simulink model "vC_3ph_MR2"  (Simulink 7.9)
settings: Solver=ode14x  StartTime=0.0  StopTime=20/60  FixedStep=Ts1  RelTol=1e-3
PostLoadFcn:
  | , if any(exist('dsrtsu_mdlpostloadfcn', 'file') == [2, 3, 6]), try dsrtsu_mdlpostloadfcn('Execute', bdroot); catch fprintf('Error in PostLoadFcn (dsrtsu_mdlpostloadfcn) for model "%s":\n %s\n', bdroot, lasterr); end, end,
InitFcn:
  | vC_ini
values from neighbouring files (symbols this model uses):
  C = Cideal+deltaC    (= 4e-05)    [IMC_calculo_limites_thetas.m]    (also in IMC_ini.m; JORGE_controlador_LCL_malha_interna.m; LCL_PAPM.m; R_in_LCL.m)
  excitacao_persistente = 0    [iC_ini.m]    (also in vC_ini.m)
  flag_time = 60/60    (= 1)    [iC_ini.m]    (also in vC_ini.m = 0)
  init_time = 60/60    (= 1)    [iC_ini.m]    (also in vC_ini.m)
  L1 = L1ideal+deltaL1    (= 0.002)    [IMC_calculo_limites_thetas.m]    (also in IMC_ini.m; LCL_PAPM.m; R_in_LCL.m; calculo_FTs.m)
  L2 = L2ideal+deltaL2+Lgideal+deltaLg    (= 0.002)    [IMC_calculo_limites_thetas.m]    (also in IMC_ini.m; LCL_PAPM.m; R_in_LCL.m; calculo_FTs.m)
  param_change_time = 60/60    (= 1)    [iC_ini.m]    (also in vC_ini.m)
  R1 = R1ideal+deltaR1    (= 1)    [IMC_calculo_limites_thetas.m]    (also in IMC_ini.m; R_in_LCL.m = 0; gera_resultados.m = 0; iC_ini.m = 0)
  R2 = R2ideal+deltaR2+Rgideal+deltaRg    (= 1)    [IMC_calculo_limites_thetas.m]    (also in IMC_ini.m; R_in_LCL.m = 0; gera_resultados.m = 0; iC_ini.m = 0)
  R_init = 10    [iC_ini.m]    (also in vC_ini.m)
  ref_phaseInv_time = 60/60    (= 1)    [iC_ini.m]    (also in vC_ini.m)
  ref_step_time = 60/60    (= 1)    [iC_ini.m]    (also in vC_ini.m)
  short_OFF_time = 61/60    (= 1.01666666667)    [vC_ini.m]
  short_ON_time = 60/60    (= 1)    [vC_ini.m]
  Ts = 0.5    [IMC_calculo_limites_thetas.m]    (also in IMC_datta_ini.m; IMC_ini.m = 8.33333333333e-05; JORGE_controlador_LCL_malha_interna.m = 8.33333333333e-05; LCL_PAPM.m = 8.33333333333e-05)
  Ts1 = Ts/10    (= 8.33333333333e-06)    [iC_ini.m]    (also in vC_ini.m)
  VCC = 1700    [iC_ini.m]    (also in vC_ini.m = 1200)
undefined symbols (not defined in the file or in its folder): D1, Delta
libraries: powerlib x38, powerlib_extras x1
(part 3 of 3)

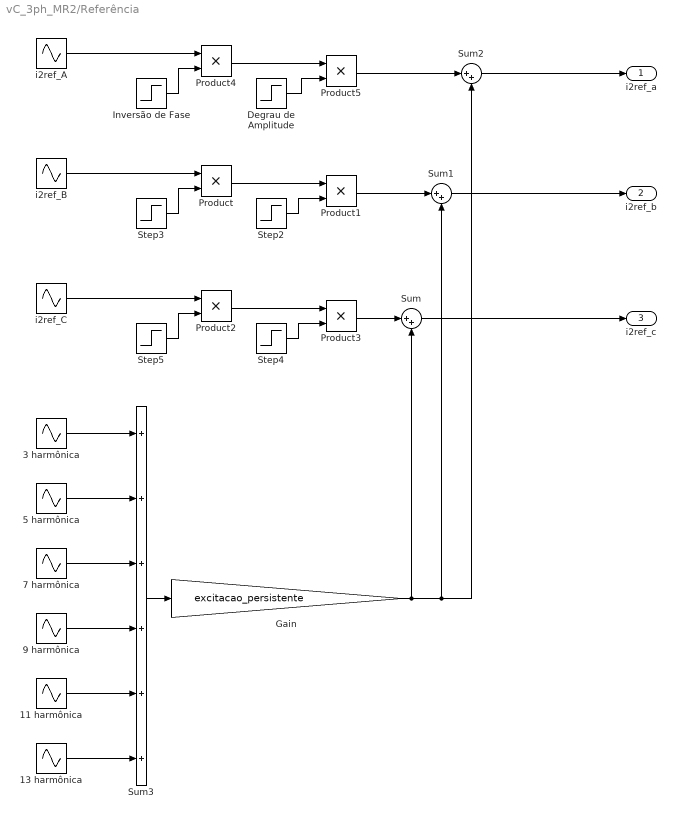
== system vC_3ph_MR2/Referência ==
  11 harmônica : Sin  Amplitude=1.2  Frequency=2*pi*60*11  SampleTime=Ts
  13 harmônica : Sin  Amplitude=1.2  Frequency=2*pi*60*13  SampleTime=Ts
  3 harmônica : Sin  Amplitude=1.2  Frequency=2*pi*60*3  SampleTime=Ts
  5 harmônica : Sin  Amplitude=1.2  Frequency=2*pi*60*5  SampleTime=Ts
  7 harmônica : Sin  Amplitude=1.2  Frequency=2*pi*60*7  SampleTime=Ts
  9 harmônica : Sin  Amplitude=1.2  Frequency=2*pi*60*9  SampleTime=Ts
  Degrau de Amplitude : Step  Time=ref_step_time  Before=1  After=2  SampleTime=Ts
  Gain : Gain  Gain=excitacao_persistente  SampleTime=Ts
  Inversão de Fase : Step  Time=ref_phaseInv_time  Before=1  After=-1  SampleTime=Ts
  Product{,1..5} (6 alike) : Product  SampleTime=Ts  RndMeth=Zero
  Step2 : Step  Time=ref_step_time  Before=1  After=2  SampleTime=Ts
  Step3 : Step  Time=ref_phaseInv_time  Before=1  After=-1  SampleTime=Ts
  Step4 : Step  Time=ref_step_time  Before=1  After=2  SampleTime=Ts
  Step5 : Step  Time=ref_phaseInv_time  Before=1  After=-1  SampleTime=Ts
  Sum : Sum  Inputs=|++
  Sum1 : Sum  Inputs=|++
  Sum2 : Sum  Inputs=|++
  Sum3 : Sum  Inputs=++++++
  i2ref_A : Sin  Amplitude=10  Frequency=2*pi*60  SampleTime=Ts
  i2ref_B : Sin  Amplitude=10  Frequency=2*pi*60  Phase=-2*pi/3  SampleTime=Ts
  i2ref_C : Sin  Amplitude=10  Frequency=2*pi*60  Phase=2*pi/3  SampleTime=Ts
  i2ref_a : Outport
  i2ref_b : Outport  Port=2
  i2ref_c : Outport  Port=3
  wires:
  Product/1 -> Product1/1
  Step3/1 -> Product/2
  Step2/1 -> Product1/2
  Product2/1 -> Product3/1
  Step5/1 -> Product2/2
  Step4/1 -> Product3/2
  Product4/1 -> Product5/1
  Inversão de Fase/1 -> Product4/2
  Degrau de Amplitude/1 -> Product5/2
  i2ref_B/1 -> Product/1
  i2ref_C/1 -> Product2/1
  i2ref_A/1 -> Product4/1
  Product5/1 -> Sum2/1
  Product1/1 -> Sum1/1
  Product3/1 -> Sum/1
  Gain/1 -> Sum/2, Sum1/2, Sum2/2
  Sum2/1 -> i2ref_a/1
  Sum1/1 -> i2ref_b/1
  Sum/1 -> i2ref_c/1
  3 harmônica/1 -> Sum3/1
  5 harmônica/1 -> Sum3/2
  7 harmônica/1 -> Sum3/3
  9 harmônica/1 -> Sum3/4
  11 harmônica/1 -> Sum3/5
  13 harmônica/1 -> Sum3/6
  Sum3/1 -> Gain/1

== matlab function Controlador/abc to alpha-beta-zero ==
  data: i2ref_a input double; i2ref_alpha output double; i2ref_b input double; i2ref_c input double; i2ref_beta output double; i2ref_0 output double
function [i2ref_alpha, i2ref_beta, i2ref_0] = abc2ab0(i2ref_a, i2ref_b, i2ref_c)
%#CODEGEN

alpha_beta_zero = [2/3 -1/3 -1/3; 0 1/sqrt(3) -1/sqrt(3); 1/3 1/3 1/3]*[i2ref_a; i2ref_b; i2ref_c];
%alpha_beta_zero = [0.66666666666667 -0.33333333333333 -0.33333333333333; 0 0.57735026918963 -0.57735026918963; 0.47140452079103 0.47140452079103 0.47140452079103]*[i2ref_a; i2ref_b; i2ref_c];

i2ref_alpha = alpha_beta_zero(1);
i2ref_beta = alpha_beta_zero(2);
i2ref_0 = alpha_beta_zero(3);

== matlab function Controlador/Controlador Adaptativo Alpha ==
  data: i2ref_k input double; up_alpha output double; i2_k input double; vc_k input double; flag input double; theta_alpha output double; t input double; m output double
function [up_alpha, theta_alpha, m] = adaptativo( i2ref_k, i2_k, vc_k, flag, t )

%#CODEGEN

%Definição dos valores projetados dos elementos do filtro
L1ideal=2e-3;
L2ideal=2e-3;
Lgideal=0;
Cideal=40e-6;
R1ideal=0;
R2ideal=0;
Rgideal=0;

%Definição de erros percentuais para simular variação paramétrica
errL1=0;
errL2=0;
errLg=0;
errC=0;
errR1=0;
errR2=0;
errRg=0;
deltaL1=errL1*L1ideal;
deltaL2=errL2*L2ideal;
deltaLg=errLg*Lgideal;
deltaC=errC*Cideal;
deltaR1=errR1*R1ideal;
deltaR2=errR2*R2ideal;
deltaRg=errRg*Rgideal;

%Definição do valor real medido, incluindo a variação paramétrica
%percentual
L1=L1ideal+deltaL1;
L2=L2ideal+deltaL2+Lgideal+deltaLg;
C=Cideal+deltaC;
R1=R1ideal+deltaR1;
R2=R2ideal+deltaR2+Rgideal+deltaRg;

%Demais elementos
Ts=1/12000;
w=sqrt((L1+L2)/(L1*L2*C));

%Kp é a multiplicação do ganho do controlador da malha interna(kp), do
%ganho da planta(ki) e do ganho da malha externa(kod)
kp_kd=3;
%Kp=0.156891976007044;
Kp=0.001792815465831;

%polos do modelo de referência:
p1=0.2;
p2=0.2;

km=(1-p1)*(1-p2);

%constantes -> gamaD < (1-gama)*km/kp
%gamaD=0.01;
gamaD=0.0098;
gama=0.99;

%delta0=0.99;
delta0=0.8;

%% Variáveis Persistentes e Inicializações

persistent theta_k;
if isempty(theta_k)
    %COM compensação para vg
    %theta_k=[-0.3106; -0.2728; 0.0368; -0.2369; -0.422; -0.2775; -0.7979; 1.786; -0.0008; 0.0003];
    %theta_k=[-0.3106; -0.2728; 0.0368; -0.2369; -0.422; -0.2775; -0.7979; 1.786; 1; 0];
    %theta_k=[-0.40085038; -0.36853743; -0.064251891; -0.4277604154; -0.61214672; -0.46675405; -0.98929343; 1.76426551; 0.17164080; 0.11598547];
    %theta_k=[0;0;0;0;0;0; -0.98929343; 1.76426551; 0.17164080; 0.11598547];
    %theta_k=[-0.071151848470510; -0.470549298500393; -0.993323557655345; 1.762541193804541; 0.118014567931226; 0.108368323169129];
    %theta_k=[-0.46; -0.58; -1.74; 1.73; 0.2; 0.03];
    theta_k=[1; -3.39; -0.18; 12.72; 1; 0];
end

persistent omega_k;
if isempty(omega_k)
    %COM vg
    omega_k=[0; 0; 0; 0; 0; 0];
end

persistent omega_k_1;
if isempty(omega_k_1)
    %COM vg
    omega_k_1=[0; 0; 0; 0; 0; 0];
end

persistent omega_k_2;
if isempty(omega_k_2)
    %COM vg
    omega_k_2=[0; 0; 0; 0; 0; 0];
end

persistent omega_k_3;
if isempty(omega_k_3)
    %COM vg
    omega_k_3=[0; 0; 0; 0; 0; 0];
end

persistent eta_k_1;
if isempty(eta_k_1)
    %COM vg
    eta_k_1=[0; 0; 0; 0; 0; 0];
end

persistent eta_k_2;
if isempty(eta_k_2)
    %COM vg
    eta_k_2=[0; 0; 0; 0; 0; 0];
end

persistent eta_k_3;
if isempty(eta_k_3)
    %COM vg
    eta_k_3=[0; 0; 0; 0; 0; 0];
end

persistent i2m_k_1;
if isempty(i2m_k_1)
    i2m_k_1=0;
end

persistent i2m_k_2;
if isempty(i2m_k_2)
    i2m_k_2=0;
end

persistent i2m_k_3;
if isempty(i2m_k_3)
    i2m_k_3=0;
end

persistent i2ref_k_1;
if isempty(i2ref_k_1)
    i2ref_k_1=0;
end

persistent i2ref_k_2;
if isempty(i2ref_k_2)
    i2ref_k_2=0;
end

persistent i2ref_k_3;
if isempty(i2ref_k_3)
    i2ref_k_3=0;
end

persistent v_k_1;
if isempty(v_k_1)
    v_k_1=0;
end

persistent v_k_2;
if isempty(v_k_2)
    v_k_2=0;
end

persistent v_k_3;
if isempty(v_k_3)
    v_k_3=0;
end

persistent rho_k;
if isempty(rho_k)
    rho_k=Kp/km;
end

persistent m2;
if isempty(m2)
    m2=1;
end

persistent vc_k_1;
if isempty(vc_k_1)
    vc_k_1=0;
end

persistent u_k_1;
if isempty(u_k_1)
    u_k_1=0;
end

persistent u_k_2;
if isempty(u_k_2)
    u_k_2=0;
end

persistent P;
if isempty(P)
    %P=[0.002225441018075 -0.002258665319558 -1.129332659782590e-004 -0.003793046611769; ...
    %    -0.002258665319558 0.149747822133961 -0.042512608892738 0.002487914954665; ...
    %    -1.129332659782590e-004 -0.042512608892738 0.997874369555398 1.243957477280539e-004; ...
    %    -0.003793046611769 0.002487914954665 1.243957477280538e-004 0.754190018333160];
    %P=[0.009712540165252   -0.000020445335620  -0.000026266935611  -0.000037334327242 -0.001161097577207  -0.000971095497459; ...
    %   -0.000020445335620   0.009977400822109  -0.000022631160072  -0.000009984284241 -0.000310511239892   0.000028021469709; ...
    %   -0.000026266935611  -0.000022631160072   0.009976301443788  -0.000009972563160 -0.000310146714255   0.000019062507239; ...
    %   -0.000037334327242  -0.000009984284241  -0.000009972563160   0.009989966652248 -0.000312037115068   0.000004936266851; ...
    %   -0.001161097577207  -0.000310511239892  -0.000310146714255  -0.000312037115068 0.000295645721395   0.000153517899078; ...
    %   -0.000971095497459   0.000028021469709   0.000019062507239   0.000004936266851 0.000153517899078   0.000171767843043];

    P=gamaD*eye(6);
end

persistent gama2;
if isempty(gama2)
    %gama2=0.997899999973786;
    gama2=gama;
end


%% Cálculos

%Ação de controle
omega_k(3)= i2_k;
omega_k(4)= i2ref_k;

%COM vg
omega_k(5)= 311*sin(2*pi*60*t);
omega_k(6)= 311*cos(2*pi*60*t);
%omega_k(5)= 0;
%omega_k(6)= 0;

u_k= theta_k'*omega_k;

%inserindo o controlador proporcional no bloco do adaptativo
up_alpha= kp_kd*(u_k - vc_k) - kp_kd*(u_k_1 - vc_k_1);

eta_k= (p1+p2)*eta_k_1 - p1*p2*eta_k_2 + (1-p1)*(1-p2)*omega_k_2;

i2m_k= (p1+p2)*i2m_k_1 - p1*p2*i2m_k_2 + (1-p1)*(1-p2)*i2ref_k_2;

e1_k= i2_k - i2m_k;

v_k= (p1+p2)*v_k_1 - p1*p2*v_k_2 + (1-p1)*(1-p2)*u_k_2;

q_k= theta_k'*eta_k;

e2_k= -v_k+q_k;

ea_k= e1_k+rho_k*e2_k;

eta2_k = eta_k;
eta2_k(5) = 0;
eta2_k(6) = 0;

if flag==1
    %m2_k= 0.01*eta_k'*eta_k + e2_k^2 + m2;
    m2_k= 0.1*eta2_k'*eta2_k + e2_k^2 + m2;
else
    %m2_k= eta_k'*eta_k + e2_k^2 + m2;
    m2_k= 0.01*eta2_k'*eta2_k + e2_k^2 + m2;
end
%m2_k= m2 + (1+eta_k'*P*eta_k) + gama2*e2_k^2;
m = m2_k;

P= P - (P*eta_k*eta_k'*P)/m2_k;
gama2= gama2 - (gama2^2*e2_k^2)/(m2_k^2);

%Pout=P;
%gama_out=gama2;

%% Atualização

%calcula theta(k+1)
theta_k = theta_k - (gamaD*ea_k/m2_k)*eta_k;
%theta_k = theta_k - (P*ea_k/m2_k)*eta_k;
theta_alpha = theta_k;

%calcula rho(k+1)
rho_k= rho_k - (gama*ea_k*e2_k)/m2_k;

if flag==1
    %m2 = delta0*(m2 - 1) + abs(u_k) + abs(i2_k) + 1;
    m2 = delta0*(m2 - 1) + abs(u_k) + abs(i2_k) + 1;
else
    %m2 = delta0*(m2 - 1) + abs(u_k)^2 + abs(i2_k)^2 + 1;
    m2 = delta0*(m2 - 1) + abs(u_k) + abs(i2_k) + 1;
end

omega_k_3=omega_k_2;
omega_k_2=omega_k_1;
omega_k_1=omega_k;

omega_k(1)=0*omega_k(1) + 1*u_k;
omega_k(2)=0*omega_k(2) + 1*i2_k;

eta_k_3=eta_k_2;
eta_k_2=eta_k_1;
eta_k_1=eta_k;

i2ref_k_3 = i2ref_k_2;
i2ref_k_2 = i2ref_k_1;
i2ref_k_1 = i2ref_k;

i2m_k_3=i2m_k_2;
i2m_k_2=i2m_k_1;
i2m_k_1=i2m_k;

v_k_3=v_k_2;
v_k_2=v_k_1;
v_k_1=v_k;

u_k_2=u_k_1;
u_k_1=u_k;

vc_k_1=vc_k;

end

== matlab function Controlador/Controlador Adaptativo Beta ==
  data: i2ref_k input double; up_beta output double; i2_k input double; vc_k input double; flag input double; t input double; theta_beta output double; m output double
function [up_beta, theta_beta, m] = adaptativo( i2ref_k, i2_k, vc_k, flag, t )

%#CODEGEN

%Definição dos valores projetados dos elementos do filtro
L1ideal=2e-3;
L2ideal=2e-3;
Lgideal=0;
Cideal=40e-6;
R1ideal=0;
R2ideal=0;
Rgideal=0;

%Definição de erros percentuais para simular variação paramétrica
errL1=0;
errL2=0;
errLg=0;
errC=0;
errR1=0;
errR2=0;
errRg=0;
deltaL1=errL1*L1ideal;
deltaL2=errL2*L2ideal;
deltaLg=errLg*Lgideal;
deltaC=errC*Cideal;
deltaR1=errR1*R1ideal;
deltaR2=errR2*R2ideal;
deltaRg=errRg*Rgideal;

%Definição do valor real medido, incluindo a variação paramétrica
%percentual
L1=L1ideal+deltaL1;
L2=L2ideal+deltaL2+Lgideal+deltaLg;
C=Cideal+deltaC;
R1=R1ideal+deltaR1;
R2=R2ideal+deltaR2+Rgideal+deltaRg;

%Demais elementos
Ts=1/12000;
w=sqrt((L1+L2)/(L1*L2*C));

%Kp é a multiplicação do ganho do controlador da malha interna(kp), do
%ganho da planta(ki) e do ganho da malha externa(kod)
kp_kd=3;
%Kp=0.156891976007044;
Kp=0.001792815465831;

%polos do modelo de referência:
p1=0.2;
p2=0.2;

km=(1-p1)*(1-p2);

%constantes -> gamaD < (1-gama)*km/kp
%gamaD=0.01;
gamaD=0.0098;
gama=0.99;

%delta0=0.99;
delta0=0.8;

%% Variáveis Persistentes e Inicializações

persistent theta_k;
if isempty(theta_k)
    %COM compensação para vg
    %theta_k=[-0.3106; -0.2728; 0.0368; -0.2369; -0.422; -0.2775; -0.7979; 1.786; -0.0008; 0.0003];
    %theta_k=[-0.3106; -0.2728; 0.0368; -0.2369; -0.422; -0.2775; -0.7979; 1.786; 1; 0];
    %theta_k=[-0.40085038; -0.36853743; -0.064251891; -0.4277604154; -0.61214672; -0.46675405; -0.98929343; 1.76426551; 0.17164080; 0.11598547];
    %theta_k=[0;0;0;0;0;0; -0.98929343; 1.76426551; 0.17164080; 0.11598547];
    %theta_k=[-0.071151848470510; -0.470549298500393; -0.993323557655345; 1.762541193804541; 0.118014567931226; 0.108368323169129];
    %theta_k=[-0.46; -0.58; -1.74; 1.73; 0.2; 0.03];
    theta_k=[1; -3.39; -0.18; 12.72; 0; 1];
end

persistent omega_k;
if isempty(omega_k)
    %COM vg
    omega_k=[0; 0; 0; 0; 0; 0];
end

persistent omega_k_1;
if isempty(omega_k_1)
    %COM vg
    omega_k_1=[0; 0; 0; 0; 0; 0];
end

persistent omega_k_2;
if isempty(omega_k_2)
    %COM vg
    omega_k_2=[0; 0; 0; 0; 0; 0];
end

persistent omega_k_3;
if isempty(omega_k_3)
    %COM vg
    omega_k_3=[0; 0; 0; 0; 0; 0];
end

persistent eta_k_1;
if isempty(eta_k_1)
    %COM vg
    eta_k_1=[0; 0; 0; 0; 0; 0];
end

persistent eta_k_2;
if isempty(eta_k_2)
    %COM vg
    eta_k_2=[0; 0; 0; 0; 0; 0];
end

persistent eta_k_3;
if isempty(eta_k_3)
    %COM vg
    eta_k_3=[0; 0; 0; 0; 0; 0];
end

persistent i2m_k_1;
if isempty(i2m_k_1)
    i2m_k_1=0;
end

persistent i2m_k_2;
if isempty(i2m_k_2)
    i2m_k_2=0;
end

persistent i2m_k_3;
if isempty(i2m_k_3)
    i2m_k_3=0;
end

persistent i2ref_k_1;
if isempty(i2ref_k_1)
    i2ref_k_1=0;
end

persistent i2ref_k_2;
if isempty(i2ref_k_2)
    i2ref_k_2=0;
end

persistent i2ref_k_3;
if isempty(i2ref_k_3)
    i2ref_k_3=0;
end

persistent v_k_1;
if isempty(v_k_1)
    v_k_1=0;
end

persistent v_k_2;
if isempty(v_k_2)
    v_k_2=0;
end

persistent v_k_3;
if isempty(v_k_3)
    v_k_3=0;
end

persistent rho_k;
if isempty(rho_k)
    rho_k=Kp/km;
end

persistent m2;
if isempty(m2)
    m2=1;
end

persistent vc_k_1;
if isempty(vc_k_1)
    vc_k_1=0;
end

persistent u_k_1;
if isempty(u_k_1)
    u_k_1=0;
end

persistent u_k_2;
if isempty(u_k_2)
    u_k_2=0;
end

persistent P;
if isempty(P)
    %P=[0.002225441018075 -0.002258665319558 -1.129332659782590e-004 -0.003793046611769; ...
    %    -0.002258665319558 0.149747822133961 -0.042512608892738 0.002487914954665; ...
    %    -1.129332659782590e-004 -0.042512608892738 0.997874369555398 1.243957477280539e-004; ...
    %    -0.003793046611769 0.002487914954665 1.243957477280538e-004 0.754190018333160];
    %P=[0.009712540165252   -0.000020445335620  -0.000026266935611  -0.000037334327242 -0.001161097577207  -0.000971095497459; ...
    %   -0.000020445335620   0.009977400822109  -0.000022631160072  -0.000009984284241 -0.000310511239892   0.000028021469709; ...
    %   -0.000026266935611  -0.000022631160072   0.009976301443788  -0.000009972563160 -0.000310146714255   0.000019062507239; ...
    %   -0.000037334327242  -0.000009984284241  -0.000009972563160   0.009989966652248 -0.000312037115068   0.000004936266851; ...
    %   -0.001161097577207  -0.000310511239892  -0.000310146714255  -0.000312037115068 0.000295645721395   0.000153517899078; ...
    %   -0.000971095497459   0.000028021469709   0.000019062507239   0.000004936266851 0.000153517899078   0.000171767843043];

    P=gamaD*eye(6);
end

persistent gama2;
if isempty(gama2)
    %gama2=0.997899999973786;
    gama2=gama;
end


%% Cálculos

%Ação de controle
omega_k(3)= i2_k;
omega_k(4)= i2ref_k;

%COM vg
omega_k(5)= 311*sin(2*pi*60*t);
omega_k(6)= 311*cos(2*pi*60*t);
%omega_k(5)= 0;
%omega_k(6)= 0;

u_k= theta_k'*omega_k;

%inserindo o controlador proporcional no bloco do adaptativo
up_beta= kp_kd*(u_k - vc_k) - kp_kd*(u_k_1 - vc_k_1);

eta_k= (p1+p2)*eta_k_1 - p1*p2*eta_k_2 + (1-p1)*(1-p2)*omega_k_2;

i2m_k= (p1+p2)*i2m_k_1 - p1*p2*i2m_k_2 + (1-p1)*(1-p2)*i2ref_k_2;

e1_k= i2_k - i2m_k;

v_k= (p1+p2)*v_k_1 - p1*p2*v_k_2 + (1-p1)*(1-p2)*u_k_2;

q_k= theta_k'*eta_k;

e2_k= -v_k+q_k;

ea_k= e1_k+rho_k*e2_k;

eta2_k = eta_k;
eta2_k(5) = 0;
eta2_k(6) = 0;

if flag==1
    %m2_k= 0.01*eta_k'*eta_k + e2_k^2 + m2;
    m2_k= 0.1*eta2_k'*eta2_k + e2_k^2 + m2;
else
    %m2_k= eta_k'*eta_k + e2_k^2 + m2;
    m2_k= 0.01*eta2_k'*eta2_k + e2_k^2 + m2;
end
%m2_k= m2 + (1+eta_k'*P*eta_k) + gama2*e2_k^2;
m = m2_k;

P= P - (P*eta_k*eta_k'*P)/m2_k;
gama2= gama2 - (gama2^2*e2_k^2)/(m2_k^2);

%Pout=P;
%gama_out=gama2;

%% Atualização

%calcula theta(k+1)
theta_k = theta_k - (gamaD*ea_k/m2_k)*eta_k;
%theta_k = theta_k - (P*ea_k/m2_k)*eta_k;
theta_beta = theta_k;

%calcula rho(k+1)
rho_k= rho_k - (gama*ea_k*e2_k)/m2_k;

if flag==1
    %m2 = delta0*(m2 - 1) + abs(u_k) + abs(i2_k) + 1;
    m2 = delta0*(m2 - 1) + abs(u_k) + abs(i2_k) + 1;
else
    %m2 = delta0*(m2 - 1) + abs(u_k)^2 + abs(i2_k)^2 + 1;
    m2 = delta0*(m2 - 1) + abs(u_k) + abs(i2_k) + 1;
end

omega_k_3=omega_k_2;
omega_k_2=omega_k_1;
omega_k_1=omega_k;

omega_k(1)=0*omega_k(1) + 1*u_k;
omega_k(2)=0*omega_k(2) + 1*i2_k;

eta_k_3=eta_k_2;
eta_k_2=eta_k_1;
eta_k_1=eta_k;

i2ref_k_3 = i2ref_k_2;
i2ref_k_2 = i2ref_k_1;
i2ref_k_1 = i2ref_k;

i2m_k_3=i2m_k_2;
i2m_k_2=i2m_k_1;
i2m_k_1=i2m_k;

v_k_3=v_k_2;
v_k_2=v_k_1;
v_k_1=v_k;

u_k_2=u_k_1;
u_k_1=u_k;

vc_k_1=vc_k;

end

== matlab function Controlador/alpha-beta-zero to abc ==
  data: up_a output double; up_alpha input double; up_b output double; up_c output double; up_beta input double; up_0 input double
function [up_a, up_b, up_c] = ab02abc(up_alpha, up_beta, up_0)
%#CODEGEN

abc = [1 0 1; -1/2 sqrt(3)/2 1; -1/2 -sqrt(3)/2 1]*[up_alpha; up_beta; up_0];
%abc= [1.00000000000000 0.00000000000000 0.70710678118655; -0.50000000000000 0.86602540378444 0.70710678118655; -0.50000000000000 -0.86602540378444 0.70710678118655]*[up_alpha; up_beta; up_0];

up_a = abc(1);
up_b = abc(2);
up_c = abc(3);

== matlab function Controlador/abc to alpha-beta-zero1 ==
  data: i2_a input double; i2_alpha output double; i2_b input double; i2_c input double; i2_beta output double; i2_0 output double
function [i2_alpha, i2_beta, i2_0] = abc2ab0(i2_a, i2_b, i2_c)
%#CODEGEN

alpha_beta_zero = [2/3 -1/3 -1/3; 0 1/sqrt(3) -1/sqrt(3); 1/3 1/3 1/3]*[i2_a; i2_b; i2_c];
%alpha_beta_zero = [0.66666666666667 -0.33333333333333 -0.33333333333333; 0 0.57735026918963 -0.57735026918963; 0.47140452079103 0.47140452079103 0.47140452079103]*[i2_a; i2_b; i2_c];

i2_alpha = alpha_beta_zero(1);
i2_beta = alpha_beta_zero(2);
i2_0 = alpha_beta_zero(3);

== matlab function Controlador/Controlador Adaptativo 0 ==
  data: i2ref_k input double; up_0 output double; i2_k input double; vc_k input double; flag input double; t input double; theta_O output double; m output double
function [up_0, theta_O, m] = adaptativo( i2ref_k, i2_k, vc_k, flag, t )

%#CODEGEN

%Definição dos valores projetados dos elementos do filtro
L1ideal=2e-3;
L2ideal=2e-3;
Lgideal=0;
Cideal=40e-6;
R1ideal=0;
R2ideal=0;
Rgideal=0;

%Definição de erros percentuais para simular variação paramétrica
errL1=0;
errL2=0;
errLg=0;
errC=0;
errR1=0;
errR2=0;
errRg=0;
deltaL1=errL1*L1ideal;
deltaL2=errL2*L2ideal;
deltaLg=errLg*Lgideal;
deltaC=errC*Cideal;
deltaR1=errR1*R1ideal;
deltaR2=errR2*R2ideal;
deltaRg=errRg*Rgideal;

%Definição do valor real medido, incluindo a variação paramétrica
%percentual
L1=L1ideal+deltaL1;
L2=L2ideal+deltaL2+Lgideal+deltaLg;
C=Cideal+deltaC;
R1=R1ideal+deltaR1;
R2=R2ideal+deltaR2+Rgideal+deltaRg;

%Demais elementos
Ts=1/12000;
w=sqrt((L1+L2)/(L1*L2*C));

%Kp é a multiplicação do ganho do controlador da malha interna(kp), do
%ganho da planta(ki) e do ganho da malha externa(kod)
kp_kd=3;
%Kp=0.156891976007044;
Kp=0.001792815465831;

%polos do modelo de referência:
p1=0.2;
p2=0.2;

km=(1-p1)*(1-p2);

%constantes -> gamaD < (1-gama)*km/kp
%gamaD=0.01;
gamaD=0.0098;
gama=0.99;

%delta0=0.99;
delta0=0.8;

%% Variáveis Persistentes e Inicializações

persistent theta_k;
if isempty(theta_k)
    %COM compensação para vg
    %theta_k=[-0.3106; -0.2728; 0.0368; -0.2369; -0.422; -0.2775; -0.7979; 1.786; -0.0008; 0.0003];
    %theta_k=[-0.3106; -0.2728; 0.0368; -0.2369; -0.422; -0.2775; -0.7979; 1.786; 1; 0];
    %theta_k=[-0.40085038; -0.36853743; -0.064251891; -0.4277604154; -0.61214672; -0.46675405; -0.98929343; 1.76426551; 0.17164080; 0.11598547];
    %theta_k=[0;0;0;0;0;0; -0.98929343; 1.76426551; 0.17164080; 0.11598547];
    %theta_k=[-0.071151848470510; -0.470549298500393; -0.993323557655345; 1.762541193804541; 0.118014567931226; 0.108368323169129];
    %theta_k=[-0.46; -0.58; -1.74; 1.73; 0.2; 0.03];
    theta_k=[1; -3.39; -0.18; 12.72; 0.07; 0.11];
end

persistent omega_k;
if isempty(omega_k)
    %COM vg
    omega_k=[0; 0; 0; 0; 0; 0];
end

persistent omega_k_1;
if isempty(omega_k_1)
    %COM vg
    omega_k_1=[0; 0; 0; 0; 0; 0];
end

persistent omega_k_2;
if isempty(omega_k_2)
    %COM vg
    omega_k_2=[0; 0; 0; 0; 0; 0];
end

persistent omega_k_3;
if isempty(omega_k_3)
    %COM vg
    omega_k_3=[0; 0; 0; 0; 0; 0];
end

persistent eta_k_1;
if isempty(eta_k_1)
    %COM vg
    eta_k_1=[0; 0; 0; 0; 0; 0];
end

persistent eta_k_2;
if isempty(eta_k_2)
    %COM vg
    eta_k_2=[0; 0; 0; 0; 0; 0];
end

persistent eta_k_3;
if isempty(eta_k_3)
    %COM vg
    eta_k_3=[0; 0; 0; 0; 0; 0];
end

persistent i2m_k_1;
if isempty(i2m_k_1)
    i2m_k_1=0;
end

persistent i2m_k_2;
if isempty(i2m_k_2)
    i2m_k_2=0;
end

persistent i2m_k_3;
if isempty(i2m_k_3)
    i2m_k_3=0;
end

persistent i2ref_k_1;
if isempty(i2ref_k_1)
    i2ref_k_1=0;
end

persistent i2ref_k_2;
if isempty(i2ref_k_2)
    i2ref_k_2=0;
end

persistent i2ref_k_3;
if isempty(i2ref_k_3)
    i2ref_k_3=0;
end

persistent v_k_1;
if isempty(v_k_1)
    v_k_1=0;
end

persistent v_k_2;
if isempty(v_k_2)
    v_k_2=0;
end

persistent v_k_3;
if isempty(v_k_3)
    v_k_3=0;
end

persistent rho_k;
if isempty(rho_k)
    rho_k=Kp/km;
end

persistent m2;
if isempty(m2)
    m2=1;
end

persistent vc_k_1;
if isempty(vc_k_1)
    vc_k_1=0;
end

persistent u_k_1;
if isempty(u_k_1)
    u_k_1=0;
end

persistent u_k_2;
if isempty(u_k_2)
    u_k_2=0;
end

persistent P;
if isempty(P)
    %P=[0.002225441018075 -0.002258665319558 -1.129332659782590e-004 -0.003793046611769; ...
    %    -0.002258665319558 0.149747822133961 -0.042512608892738 0.002487914954665; ...
    %    -1.129332659782590e-004 -0.042512608892738 0.997874369555398 1.243957477280539e-004; ...
    %    -0.003793046611769 0.002487914954665 1.243957477280538e-004 0.754190018333160];
    %P=[0.009712540165252   -0.000020445335620  -0.000026266935611  -0.000037334327242 -0.001161097577207  -0.000971095497459; ...
    %   -0.000020445335620   0.009977400822109  -0.000022631160072  -0.000009984284241 -0.000310511239892   0.000028021469709; ...
    %   -0.000026266935611  -0.000022631160072   0.009976301443788  -0.000009972563160 -0.000310146714255   0.000019062507239; ...
    %   -0.000037334327242  -0.000009984284241  -0.000009972563160   0.009989966652248 -0.000312037115068   0.000004936266851; ...
    %   -0.001161097577207  -0.000310511239892  -0.000310146714255  -0.000312037115068 0.000295645721395   0.000153517899078; ...
    %   -0.000971095497459   0.000028021469709   0.000019062507239   0.000004936266851 0.000153517899078   0.000171767843043];

    P=gamaD*eye(6);
end

persistent gama2;
if isempty(gama2)
    %gama2=0.997899999973786;
    gama2=gama;
end


%% Cálculos

%Ação de controle
omega_k(3)= i2_k;
omega_k(4)= i2ref_k;

%COM vg
omega_k(5)= 311*sin(2*pi*60*t);
omega_k(6)= 311*cos(2*pi*60*t);
%omega_k(5)= 0;
%omega_k(6)= 0;

u_k= theta_k'*omega_k;

%inserindo o controlador proporcional no bloco do adaptativo
up_0= kp_kd*(u_k - vc_k) - kp_kd*(u_k_1 - vc_k_1);

eta_k= (p1+p2)*eta_k_1 - p1*p2*eta_k_2 + (1-p1)*(1-p2)*omega_k_2;

i2m_k= (p1+p2)*i2m_k_1 - p1*p2*i2m_k_2 + (1-p1)*(1-p2)*i2ref_k_2;

e1_k= i2_k - i2m_k;

v_k= (p1+p2)*v_k_1 - p1*p2*v_k_2 + (1-p1)*(1-p2)*u_k_2;

q_k= theta_k'*eta_k;

e2_k= -v_k+q_k;

ea_k= e1_k+rho_k*e2_k;

eta2_k = eta_k;
eta2_k(5) = 0;
eta2_k(6) = 0;

if flag==1
    %m2_k= 0.01*eta_k'*eta_k + e2_k^2 + m2;
    m2_k= 0.1*eta2_k'*eta2_k + e2_k^2 + m2;
else
    %m2_k= eta_k'*eta_k + e2_k^2 + m2;
    m2_k= 0.01*eta2_k'*eta2_k + e2_k^2 + m2;
end
%m2_k= m2 + (1+eta_k'*P*eta_k) + gama2*e2_k^2;
m = m2_k;

P= P - (P*eta_k*eta_k'*P)/m2_k;
gama2= gama2 - (gama2^2*e2_k^2)/(m2_k^2);

%Pout=P;
%gama_out=gama2;

%% Atualização

%calcula theta(k+1)
theta_k = theta_k - (gamaD*ea_k/m2_k)*eta_k;
%theta_k = theta_k - (P*ea_k/m2_k)*eta_k;
theta_O = theta_k;

%calcula rho(k+1)
rho_k= rho_k - (gama*ea_k*e2_k)/m2_k;

if flag==1
    %m2 = delta0*(m2 - 1) + abs(u_k) + abs(i2_k) + 1;
    m2 = delta0*(m2 - 1) + abs(u_k) + abs(i2_k) + 1;
else
    %m2 = delta0*(m2 - 1) + abs(u_k)^2 + abs(i2_k)^2 + 1;
    m2 = delta0*(m2 - 1) + abs(u_k) + abs(i2_k) + 1;
end

omega_k_3=omega_k_2;
omega_k_2=omega_k_1;
omega_k_1=omega_k;

omega_k(1)=0*omega_k(1) + 1*u_k;
omega_k(2)=0*omega_k(2) + 1*i2_k;

eta_k_3=eta_k_2;
eta_k_2=eta_k_1;
eta_k_1=eta_k;

i2ref_k_3 = i2ref_k_2;
i2ref_k_2 = i2ref_k_1;
i2ref_k_1 = i2ref_k;

i2m_k_3=i2m_k_2;
i2m_k_2=i2m_k_1;
i2m_k_1=i2m_k;

v_k_3=v_k_2;
v_k_2=v_k_1;
v_k_1=v_k;

u_k_2=u_k_1;
u_k_1=u_k;

vc_k_1=vc_k;

end

== matlab function Controlador/abc to alpha-beta-zero2 ==
  data: vC_a input double; vC_alpha output double; vC_b input double; vC_c input double; vC_beta output double; vC_0 output double
function [vC_alpha, vC_beta, vC_0] = abc2ab0(vC_a, vC_b, vC_c)
%#CODEGEN

alpha_beta_zero = [2/3 -1/3 -1/3; 0 1/sqrt(3) -1/sqrt(3); 1/3 1/3 1/3]*[vC_a; vC_b; vC_c];
%alpha_beta_zero = [0.66666666666667 -0.33333333333333 -0.33333333333333; 0 0.57735026918963 -0.57735026918963; 0.47140452079103 0.47140452079103 0.47140452079103]*[iC_a; iC_b; iC_c];

vC_alpha = alpha_beta_zero(1);
vC_beta = alpha_beta_zero(2);
vC_0 = alpha_beta_zero(3);
